simulink model "drone_discrete"  (R2020b)
settings: Solver=VariableStepAuto  StartTime=0.0  StopTime=1  FixedStep=0.005  MaxStep=1e-5  MinStep=1e-8  RelTol=1e-3
values from neighbouring files (symbols this model uses):
  AttDyna_Ixx = 0.0211    [make.m]
  AttDyna_Iyy = 0.0219    [make.m]
  AttDyna_Izz = 0.0366    [make.m]
  ConEfficiency_drone_cM = 1.779e-07    [make.m]
  ConEfficiency_drone_cT = 1.105e-05    [make.m]
  ConEfficiency_drone_R = 0.225    [make.m]
  PosDyna_GravityAcc = 9.8    [make.m]
  PosDyna_Mass = 1.4    [make.m]
  PowerUnit_CR = 1148    [make.m]
  PowerUnit_Tm = 0.02    [make.m]
  PowerUnit_wb = -141.4    [make.m]
settings Model: Creator=ZhangZheng  LastModifiedBy=ASUS
settings DataIOCC: ReturnWorkspaceOutputs=off
settings DebuggingCC: ArithmeticOperatorsInVariantConditions=warning
settings SFSimCC: SimUseLocalCustomCode=off  CustomCodeUndefinedFunction=UseInterfaceOnly
settings RTWCC: RTWUseLocalCustomCode=off

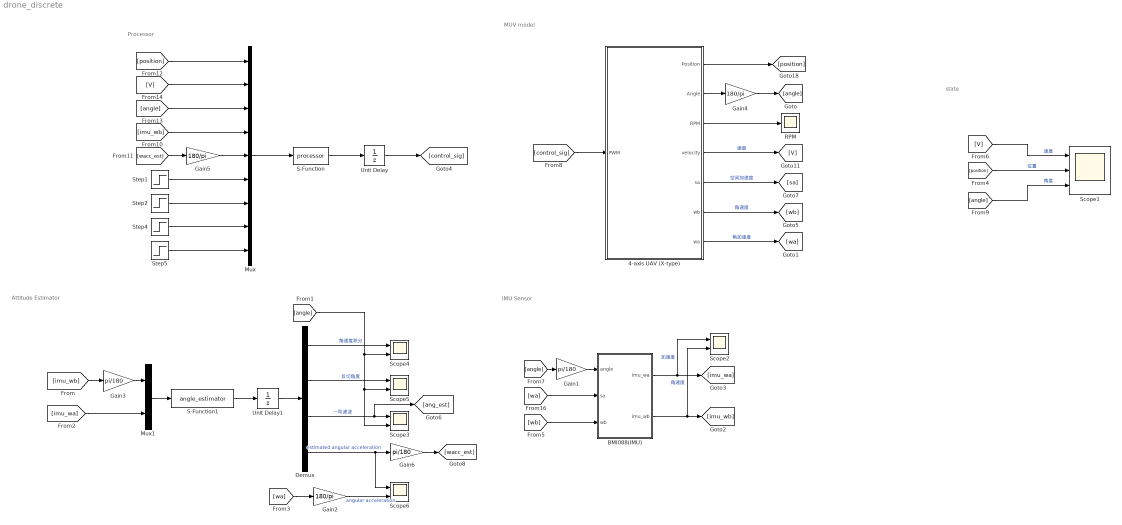
== system drone_discrete ==
  note: Attitude Estimator
  note: state
  note: MUV model
  note: Processor
  note: IMU Sensor
  4-axis UAV (X-type) : Subsystem
  BMI088(IMU) : Subsystem
  Demux : Demux
  Gain1 : Gain  Gain=pi/180
  Gain2 : Gain  Gain=180/pi
  Gain3 : Gain  Gain=pi/180
  Gain4 : Gain  Gain=180/pi
  Gain5 : Gain  Gain=180/pi
  Gain6 : Gain  Gain=pi/180
  Mux : Mux  Inputs=9
  Mux1 : Mux  Inputs=2
  RPM : Scope
  S-Function : S-Function  FunctionName=processor  SFunctionDeploymentMode=off  EnableBusSupport=off
  S-Function1 : S-Function  FunctionName=angle_estimator  SFunctionDeploymentMode=off  EnableBusSupport=off
  Scope1 : Scope  NumInputPorts=3
  Scope{2..6} (5 alike) : Scope  NumInputPorts=2
  Step1 : Step  Time=0  After=0  SampleTime=0
  Step2 : Step  Time=10  After=0  SampleTime=0
  Step4 : Step  Time=20  After=0*pi/180  SampleTime=0
  Step5 : Step  Time=0  After=0  SampleTime=0
  Unit Delay : UnitDelay  SampleTime=-1  HasFrameUpgradeWarning=on
  Unit Delay1 : UnitDelay  SampleTime=-1  HasFrameUpgradeWarning=on
  wires:
  4-axis UAV (X-type)/2(Angle) -> Gain4/1
  4-axis UAV (X-type)/3(RPM) -> RPM/1
  4-axis UAV (X-type)/1(Position) -> [position]
  4-axis UAV (X-type)/4(velocity) -> [V]  "速度"
  4-axis UAV (X-type)/6(wb) -> [wb]  "角速度"
  Mux/1 -> S-Function/1
  [V] -> Mux/2
  [position] -> Mux/1
  S-Function/1 -> Unit Delay/1
  Mux1/1 -> S-Function1/1
  [imu_wb] -> Gain3/1
  [imu_wa] -> Mux1/2
  S-Function1/1 -> Unit Delay1/1
  [V] -> Scope1/1  "速度"
  [position] -> Scope1/2  "位置"
  BMI088(IMU)/1(imu_wa) -> Scope2/1, [imu_wa]  "加速度"
  [wa] -> BMI088(IMU)/2(sa)
  [wb] -> BMI088(IMU)/3(wb)
  BMI088(IMU)/2(imu_wb) -> [imu_wb], Scope2/2  "角速度"
  Unit Delay/1 -> [control_sig]
  [control_sig] -> 4-axis UAV (X-type)/1(PWM)
  [angle] -> Scope1/3  "角度"
  Unit Delay1/1 -> Demux/1
  [imu_wb] -> Mux/4
  4-axis UAV (X-type)/5(sa) -> [sa]  "空间加速度"
  4-axis UAV (X-type)/7(wa) -> [wa]  "角加速度"
  [angle] -> Mux/3
  Gain4/1 -> [angle]
  [angle] -> Gain1/1
  Gain1/1 -> BMI088(IMU)/1(angle)
  Demux/1 -> Scope4/1  "角速度积分"
  Demux/3 -> [ang_est], Scope3/1  "一阶滤波"
  Demux/2 -> Scope5/1  "反切角度"
  [angle] -> Scope3/2, Scope5/2, Scope4/2
  Demux/4 -> Gain6/1, Scope6/1  "estimated angular acceleration"
  Step5/1 -> Mux/9
  Step4/1 -> Mux/8
  Step2/1 -> Mux/7
  Step1/1 -> Mux/6
  Gain3/1 -> Mux1/1
  [wacc_est] -> Gain5/1
  [wa] -> Gain2/1
  Gain2/1 -> Scope6/2  "angular acceleration"
  Gain5/1 -> Mux/5
  Gain6/1 -> [wacc_est]

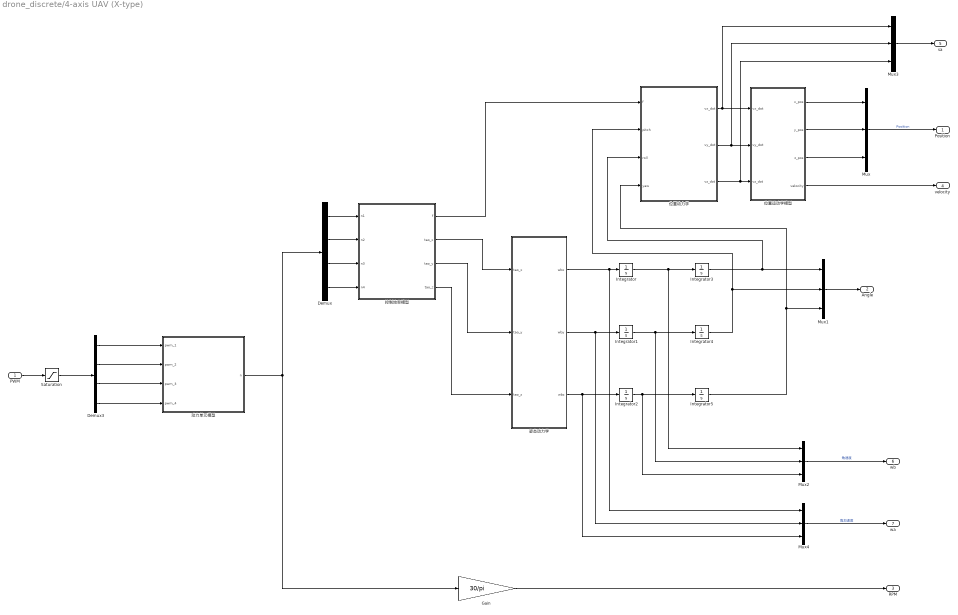
== system drone_discrete/4-axis UAV (X-type) ==
  PWM : Inport
  Demux : Demux
  Demux3 : Demux
  Gain : Gain  Gain=30/pi
  Integrator{,1..5} (6 alike) : Integrator
  Mux{,1..4} (5 alike) : Mux  Inputs=3
  Saturation : Saturate  UpperLimit=1  LowerLimit=0
  位置动力学 : Subsystem
  位置运动学模型 : Subsystem
  动力单元模型 : Subsystem
  姿态动力学 : Subsystem
  控制效率模型 : Subsystem
  Position : Outport
  Angle : Outport  Port=2
  RPM : Outport  Port=3
  velocity : Outport  Port=4
  sa : Outport  Port=5
  wb : Outport  Port=6
  wa : Outport  Port=7
  wires:
  控制效率模型/3(tao_y) -> 姿态动力学/2(tao_y)
  Demux/2 -> 控制效率模型/2(n2)
  控制效率模型/1(f) -> 位置动力学/1(f)
  位置动力学/3(vz_dot) -> Mux3/3, 位置运动学模型/3(vz_dot)
  控制效率模型/2(tao_x) -> 姿态动力学/1(tao_x)
  Integrator4/1 -> Mux1/2, 位置动力学/2(pitch)
  位置动力学/1(vx_dot) -> 位置运动学模型/1(vx_dot), Mux3/1
  Mux/1 -> Position/1  "Position"
  Demux/4 -> 控制效率模型/4(n4)
  Gain/1 -> RPM/1
  位置运动学模型/3(z_pos) -> Mux/3
  Integrator5/1 -> Mux1/3, 位置动力学/4(yaw)
  Integrator3/1 -> Mux1/1, 位置动力学/3(roll)
  Demux/3 -> 控制效率模型/3(n3)
  Demux/1 -> 控制效率模型/1(n1)
  控制效率模型/4(tao_z) -> 姿态动力学/3(tao_z)
  姿态动力学/2(wby) -> Mux4/2, Integrator1/1
  位置运动学模型/1(x_pos) -> Mux/1
  PWM/1 -> Saturation/1
  动力单元模型/1(n) -> Demux/1, Gain/1
  位置运动学模型/2(y_pos) -> Mux/2
  位置动力学/2(vy_dot) -> Mux3/2, 位置运动学模型/2(vy_dot)
  Mux1/1 -> Angle/1
  姿态动力学/1(wbx) -> Mux4/1, Integrator/1
  Mux2/1 -> wb/1  "角速度"
  位置运动学模型/4(velocity) -> velocity/1
  Saturation/1 -> Demux3/1
  Integrator/1 -> Mux2/1, Integrator3/1
  Integrator1/1 -> Integrator4/1, Mux2/2
  姿态动力学/3(wbz) -> Mux4/3, Integrator2/1
  Integrator2/1 -> Integrator5/1, Mux2/3
  Mux3/1 -> sa/1
  Mux4/1 -> wa/1  "角加速度"
  Demux3/4 -> 动力单元模型/4(pwm_4)
  Demux3/3 -> 动力单元模型/3(pwm_3)
  Demux3/2 -> 动力单元模型/2(pwm_2)
  Demux3/1 -> 动力单元模型/1(pwm_1)

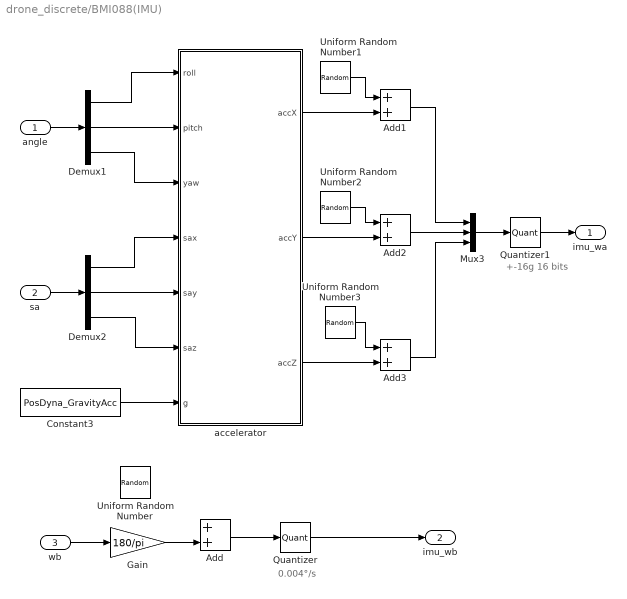
== system drone_discrete/BMI088(IMU) ==
  note: 0.004°/s
  note: +-16g
      | 16 bits
  angle : Inport
  sa : Inport  Port=2
  wb : Inport  Port=3
  Add{,1..3} (4 alike) : Sum
  Constant3 : Constant  Value=PosDyna_GravityAcc
  Demux1 : Demux  Outputs=3
  Demux2 : Demux  Outputs=3
  Gain : Gain  Gain=180/pi
  Mux3 : Mux  Inputs=3
  Quantizer : Quantizer  QuantizationInterval=0.004*pi/180
  Quantizer1 : Quantizer  QuantizationInterval=32*9.8/(2^16-1)
  Uniform Random Number : UniformRandomNumber  SampleTime=1/1000
  Uniform Random Number1 : UniformRandomNumber  Minimum=-0.5  Maximum=0.5  SampleTime=1/100
  Uniform Random Number2 : UniformRandomNumber  Minimum=-0.5  Maximum=0.5  SampleTime=1/100
  Uniform Random Number3 : UniformRandomNumber  Minimum=-0.5  Maximum=0.5  SampleTime=1/100
  accelerator : MATLAB Function  TreatAsAtomicUnit=on
  imu_wa : Outport
  imu_wb : Outport  Port=2
  wires:
  Demux1/3 -> accelerator/3(yaw)
  Demux1/1 -> accelerator/1(roll)
  Demux1/2 -> accelerator/2(pitch)
  angle/1 -> Demux1/1
  Mux3/1 -> Quantizer1/1
  Quantizer1/1 -> imu_wa/1
  Quantizer/1 -> imu_wb/1
  Add/1 -> Quantizer/1
  wb/1 -> Gain/1
  accelerator/1(accX) -> Add1/2
  Add1/1 -> Mux3/1
  accelerator/2(accY) -> Add2/2
  accelerator/3(accZ) -> Add3/2
  Add2/1 -> Mux3/2
  Add3/1 -> Mux3/3
  Gain/1 -> Add/2
  sa/1 -> Demux2/1
  Demux2/1 -> accelerator/4(sax)
  Demux2/2 -> accelerator/5(say)
  Demux2/3 -> accelerator/6(saz)
  Constant3/1 -> accelerator/7(g)
  Uniform Random Number2/1 -> Add2/1
  Uniform Random Number3/1 -> Add3/1
  Uniform Random Number1/1 -> Add1/1

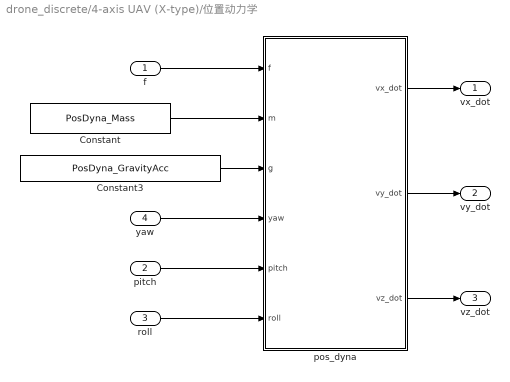
== system drone_discrete/4-axis UAV (X-type)/位置动力学 ==
  f : Inport
  pitch : Inport  Port=2
  roll : Inport  Port=3
  yaw : Inport  Port=4
  Constant : Constant  Value=PosDyna_Mass
  Constant3 : Constant  Value=PosDyna_GravityAcc
  pos_dyna : MATLAB Function  TreatAsAtomicUnit=on
  vx_dot : Outport  VectorParamsAs1DForOutWhenUnconnected=off
  vy_dot : Outport  Port=2  VectorParamsAs1DForOutWhenUnconnected=off
  vz_dot : Outport  Port=3  VectorParamsAs1DForOutWhenUnconnected=off
  wires:
  pos_dyna/1(vx_dot) -> vx_dot/1
  Constant/1 -> pos_dyna/2(m)
  pos_dyna/3(vz_dot) -> vz_dot/1
  pos_dyna/2(vy_dot) -> vy_dot/1
  Constant3/1 -> pos_dyna/3(g)
  yaw/1 -> pos_dyna/4(yaw)
  pitch/1 -> pos_dyna/5(pitch)
  roll/1 -> pos_dyna/6(roll)
  f/1 -> pos_dyna/1(f)

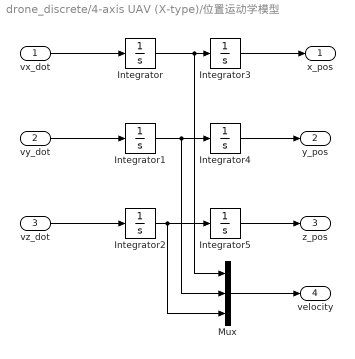
== system drone_discrete/4-axis UAV (X-type)/位置运动学模型 ==
  vx_dot : Inport
  vy_dot : Inport  Port=2
  vz_dot : Inport  Port=3
  Integrator{,1..5} (6 alike) : Integrator
  Mux : Mux  Inputs=3
  x_pos : Outport  VectorParamsAs1DForOutWhenUnconnected=off
  y_pos : Outport  Port=2  VectorParamsAs1DForOutWhenUnconnected=off
  z_pos : Outport  Port=3  VectorParamsAs1DForOutWhenUnconnected=off
  velocity : Outport  Port=4
  wires:
  Integrator1/1 -> Mux/2, Integrator4/1
  Integrator/1 -> Mux/1, Integrator3/1
  Integrator2/1 -> Mux/3, Integrator5/1
  vz_dot/1 -> Integrator2/1
  Integrator5/1 -> z_pos/1
  vx_dot/1 -> Integrator/1
  vy_dot/1 -> Integrator1/1
  Integrator4/1 -> y_pos/1
  Integrator3/1 -> x_pos/1
  Mux/1 -> velocity/1

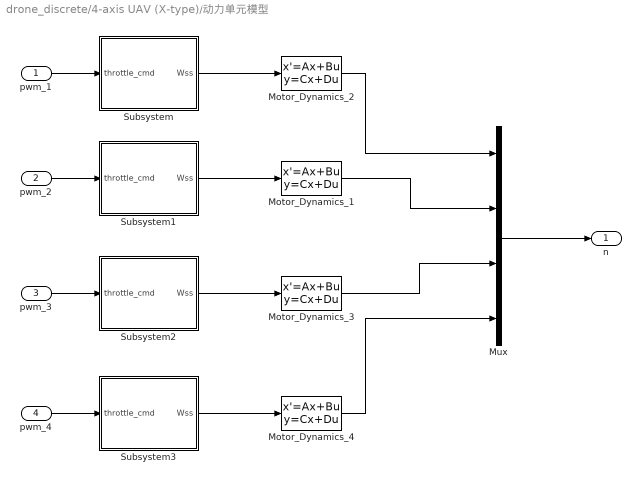
== system drone_discrete/4-axis UAV (X-type)/动力单元模型 ==
  pwm_1 : Inport
  pwm_2 : Inport  Port=2
  pwm_3 : Inport  Port=3
  pwm_4 : Inport  Port=4
  Motor_Dynamics_{1..4} (4 alike) : StateSpace  A=-1/PowerUnit_Tm  C=1/PowerUnit_Tm  D=0  InitialCondition=557.142*PowerUnit_Tm
  Mux : Mux
  Subsystem : Subsystem
  Subsystem1 : Subsystem
  Subsystem2 : Subsystem
  Subsystem3 : Subsystem
  n : Outport  VectorParamsAs1DForOutWhenUnconnected=off
  wires:
  pwm_4/1 -> Subsystem3/1("throttle_cmd ")
  pwm_2/1 -> Subsystem1/1("throttle_cmd ")
  Subsystem2/1(Wss) -> Motor_Dynamics_3/1
  Mux/1 -> n/1
  Subsystem1/1(Wss) -> Motor_Dynamics_1/1
  pwm_3/1 -> Subsystem2/1("throttle_cmd ")
  Motor_Dynamics_4/1 -> Mux/4
  Subsystem3/1(Wss) -> Motor_Dynamics_4/1
  Motor_Dynamics_2/1 -> Mux/1
  pwm_1/1 -> Subsystem/1("throttle_cmd ")
  Motor_Dynamics_3/1 -> Mux/3
  Subsystem/1(Wss) -> Motor_Dynamics_2/1
  Motor_Dynamics_1/1 -> Mux/2

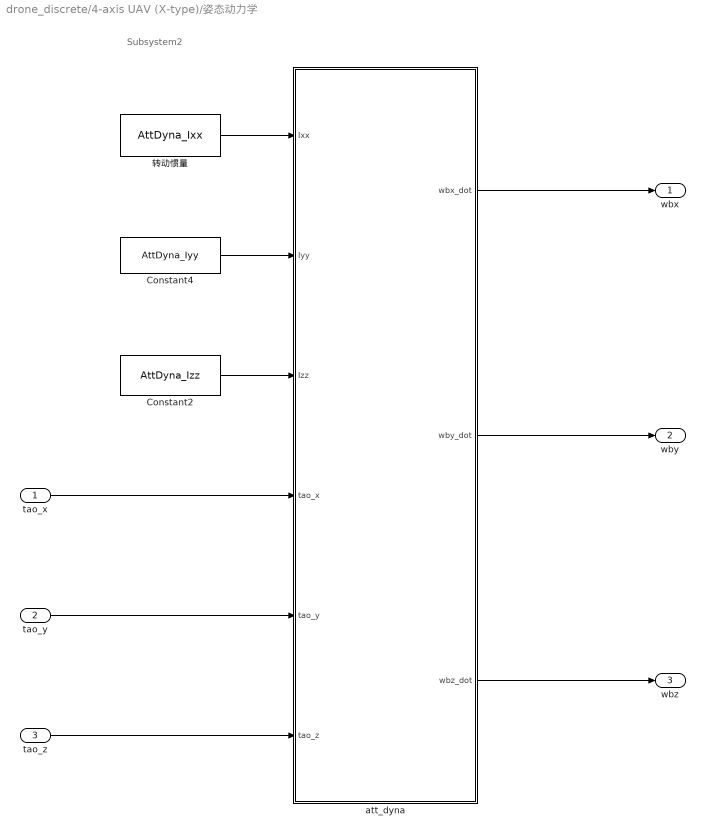
== system drone_discrete/4-axis UAV (X-type)/姿态动力学 ==
  note: Subsystem2
  tao_x : Inport
  tao_y : Inport  Port=2
  tao_z : Inport  Port=3
  Constant2 : Constant  Value=AttDyna_Izz
  Constant4 : Constant  Value=AttDyna_Iyy
  att_dyna : MATLAB Function  TreatAsAtomicUnit=on
  转动惯量 : Constant  Value=AttDyna_Ixx
  wbx : Outport  VectorParamsAs1DForOutWhenUnconnected=off
  wby : Outport  Port=2  VectorParamsAs1DForOutWhenUnconnected=off
  wbz : Outport  Port=3  VectorParamsAs1DForOutWhenUnconnected=off
  wires:
  tao_y/1 -> att_dyna/5(tao_y)
  tao_z/1 -> att_dyna/6(tao_z)
  tao_x/1 -> att_dyna/4(tao_x)
  att_dyna/3(wbz_dot) -> wbz/1
  att_dyna/1(wbx_dot) -> wbx/1
  att_dyna/2(wby_dot) -> wby/1
  Constant2/1 -> att_dyna/3(Izz)
  Constant4/1 -> att_dyna/2(Iyy)
  转动惯量/1 -> att_dyna/1(Ixx)

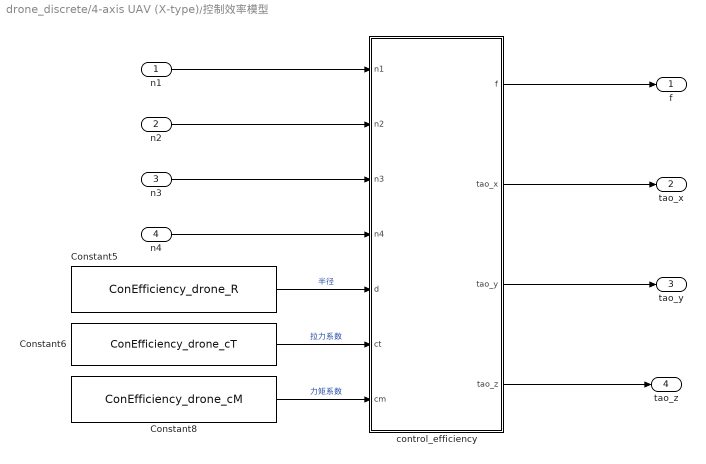
== system drone_discrete/4-axis UAV (X-type)/控制效率模型 ==
  n1 : Inport
  n2 : Inport  Port=2
  n3 : Inport  Port=3
  n4 : Inport  Port=4
  Constant5 : Constant  Value=ConEfficiency_drone_R
  Constant6 : Constant  Value=ConEfficiency_drone_cT
  Constant8 : Constant  Value=ConEfficiency_drone_cM
  control_efficiency : MATLAB Function  TreatAsAtomicUnit=on
  f : Outport  VectorParamsAs1DForOutWhenUnconnected=off
  tao_x : Outport  Port=2  VectorParamsAs1DForOutWhenUnconnected=off
  tao_y : Outport  Port=3  VectorParamsAs1DForOutWhenUnconnected=off
  tao_z : Outport  Port=4  VectorParamsAs1DForOutWhenUnconnected=off
  wires:
  control_efficiency/1(f) -> f/1
  control_efficiency/4(tao_z) -> tao_z/1
  n4/1 -> control_efficiency/4(n4)
  control_efficiency/2(tao_x) -> tao_x/1
  n3/1 -> control_efficiency/3(n3)
  control_efficiency/3(tao_y) -> tao_y/1
  n2/1 -> control_efficiency/2(n2)
  Constant8/1 -> control_efficiency/7(cm)  "力矩系数"
  n1/1 -> control_efficiency/1(n1)
  Constant5/1 -> control_efficiency/5(d)  "半径"
  Constant6/1 -> control_efficiency/6(ct)  "拉力系数"

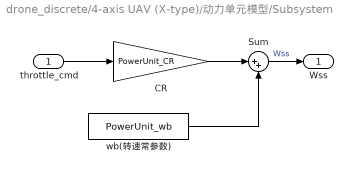
== system drone_discrete/4-axis UAV (X-type)/动力单元模型/Subsystem ==
  "throttle_cmd " : Inport
  CR : Gain  Gain=PowerUnit_CR
  Sum : Sum  Inputs=|++
  wb(转速常参数) : Constant  Value=PowerUnit_wb
  Wss : Outport  VectorParamsAs1DForOutWhenUnconnected=off
  wires:
  "throttle_cmd "/1 -> CR/1
  CR/1 -> Sum/1
  wb(转速常参数)/1 -> Sum/2
  Sum/1 -> Wss/1  "Wss"

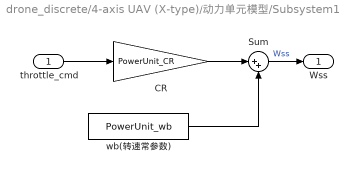
== system drone_discrete/4-axis UAV (X-type)/动力单元模型/Subsystem1 ==
  "throttle_cmd " : Inport
  CR : Gain  Gain=PowerUnit_CR
  Sum : Sum  Inputs=|++
  wb(转速常参数) : Constant  Value=PowerUnit_wb
  Wss : Outport  VectorParamsAs1DForOutWhenUnconnected=off
  wires:
  Sum/1 -> Wss/1  "Wss"
  wb(转速常参数)/1 -> Sum/2
  CR/1 -> Sum/1
  "throttle_cmd "/1 -> CR/1

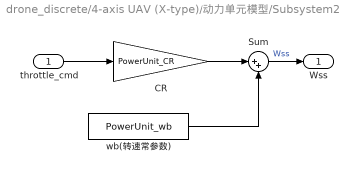
== system drone_discrete/4-axis UAV (X-type)/动力单元模型/Subsystem2 ==
  "throttle_cmd " : Inport
  CR : Gain  Gain=PowerUnit_CR
  Sum : Sum  Inputs=|++
  wb(转速常参数) : Constant  Value=PowerUnit_wb
  Wss : Outport  VectorParamsAs1DForOutWhenUnconnected=off
  wires:
  "throttle_cmd "/1 -> CR/1
  CR/1 -> Sum/1
  wb(转速常参数)/1 -> Sum/2
  Sum/1 -> Wss/1  "Wss"

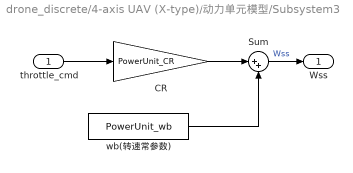
== system drone_discrete/4-axis UAV (X-type)/动力单元模型/Subsystem3 ==
  "throttle_cmd " : Inport
  CR : Gain  Gain=PowerUnit_CR
  Sum : Sum  Inputs=|++
  wb(转速常参数) : Constant  Value=PowerUnit_wb
  Wss : Outport  VectorParamsAs1DForOutWhenUnconnected=off
  wires:
  Sum/1 -> Wss/1  "Wss"
  wb(转速常参数)/1 -> Sum/2
  CR/1 -> Sum/1
  "throttle_cmd "/1 -> CR/1

== matlab function drone_discrete/BMI088(IMU)/accelerator ==
  data: roll input; pitch input; yaw input; sax input; say input; saz input; accX output; g input; accY output; accZ output
function [accX, accY, accZ]            = accelerator(roll,pitch,yaw,sax,say,saz,g)

accX = -sin(pitch)*cos(roll)*(g+saz); 
accX = accX + (cos(pitch)*cos(yaw)+sin(pitch)*sin(roll)*sin(yaw))*sax; 
accX = accX + (sin(pitch)*cos(yaw)*sin(roll)-cos(pitch)*sin(yaw))*say;

accY = sin(roll)*(g+saz);
accY = accY + sin(yaw)*cos(roll)*sax;
accY = accY + cos(yaw)*cos(roll)*say;
        
accZ = cos(pitch)*cos(roll)*(g+saz);
accZ = accZ + (sin(pitch)*cos(yaw)-cos(pitch)*sin(yaw)*sin(roll))*sax;
accZ = accZ + (-sin(pitch)*sin(yaw)-cos(pitch)*cos(yaw)*sin(roll))*say;          


end

== matlab function drone_discrete/4-axis UAV (X-type)/位置动力学/pos_dyna ==
  data: f input; vx_dot output; m input; g input; yaw input; pitch input; roll input; vy_dot output; vz_dot output
function [vx_dot,vy_dot,vz_dot] = pos_dyna(f,m,g,yaw,pitch,roll)
%输入：拉力，重力，三个欧拉角
%输出：空间坐标系下的三个加速度
vx_dot = (sin(roll)*sin(yaw) + cos(roll)*cos(yaw)*sin(pitch))*f/m;
vy_dot = (cos(roll)*sin(pitch)*sin(yaw) - cos(yaw)*sin(roll))*f/m;
vz_dot = (cos(pitch)*cos(roll)*f/m)+g;
end

== matlab function drone_discrete/4-axis UAV (X-type)/姿态动力学/att_dyna ==
  data: Ixx input; Iyy input; Izz input; tao_x input; tao_y input; tao_z input; wbx_dot output; wby_dot output; wbz_dot output
function [wbx_dot,wby_dot,wbz_dot] = att_dyna(Ixx,Iyy,Izz,tao_x,tao_y,tao_z)
% wb = [wbx wby wbz]';
% wb_cha = [   0 -wbz   wby;
%            wbz    0  -wbx;
%           -wby  wbx     0];
% I = [Ixx   0   0;
%        0 Iyy   0;
%        0   0 Izz];
I_inv = [1/Ixx     0     0; %转动惯量
             0 1/Iyy     0;
             0     0 1/Izz];
tao = [tao_x tao_y tao_z]';
% G_x = Jrp * wby * (n1+n2-n3-n4);
% G_y = Jrp * wbx * (-n1-n2+n3+n4);
% G_z = 0;  
% G = [G_x G_y G_z]';
wb_dot = I_inv * (tao);
wbx_dot = wb_dot(1,1);
wby_dot = wb_dot(2,1);  
wbz_dot = wb_dot(3,1);
end

== matlab function drone_discrete/4-axis UAV (X-type)/控制效率模型/control_efficiency ==
  data: n1 input; f output; n2 input; n3 input; n4 input; tao_x output; tao_y output; tao_z output; d input; ct input; cm input
function [f,tao_x,tao_y,tao_z] = control_efficiency(n1,n2,n3,n4,d,ct,cm)
%控制效率模型
%X型机架
%3↓   1↑
%  \ /
%  / \
%2↑   4↓
%转速单位是弧度/s
f = -1*ct*(n1^2 + n2^2 + n3^2 + n4^2);%z轴朝下，所以拉力为负
tao_x = d*ct*sin(pi/4)*(-n1^2 + n2^2 + n3^2 - n4^2) / 2;
tao_y = d*ct*sin(pi/4)*(n1^2 - n2^2 + n3^2 - n4^2) / 2;
tao_z = cm*(n1^2 + n2^2 - n3^2 - n4^2);     %旋转力矩
%十字型
% f = ct*(n1^2 + n2^2 + n3^2 + n4^2);
% tao_x = -d*ct*n2^2 + d*ct*n4^2;
% tao_y =  d*ct*n1^2 - d*ct*n3^2;
% tao_z = cm*(n1^2 - n2^2 + n3^2 - n4^2);
end
